simulink model "planLocal_sim"  (R2024a)
settings: Solver=FixedStepDiscrete  StartTime=0.0  StopTime=30  RelTol=1e-3
InitFcn:
  | localPlanSetup
undefined symbols (not defined in the file): n, refPath, tuneableTEBParamsCpp, worldGridLoc, worldMat, worldRes
libraries: roshelperlib x2, simulink x1
settings Model: Creator=cstabile  LastModifiedBy=cstabile
settings SFSimCC: SimTargetLang=C++

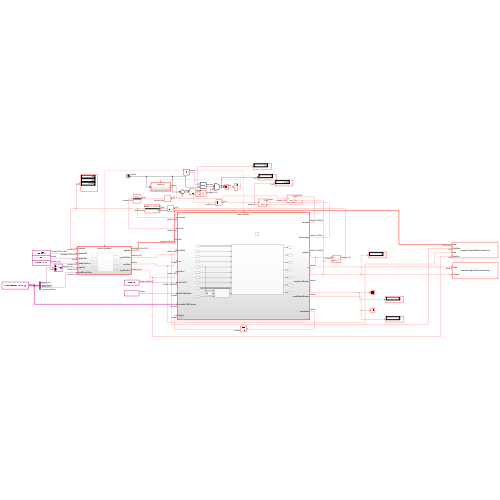
[thumbnail: Simulink's stored preview of the top-level diagram]
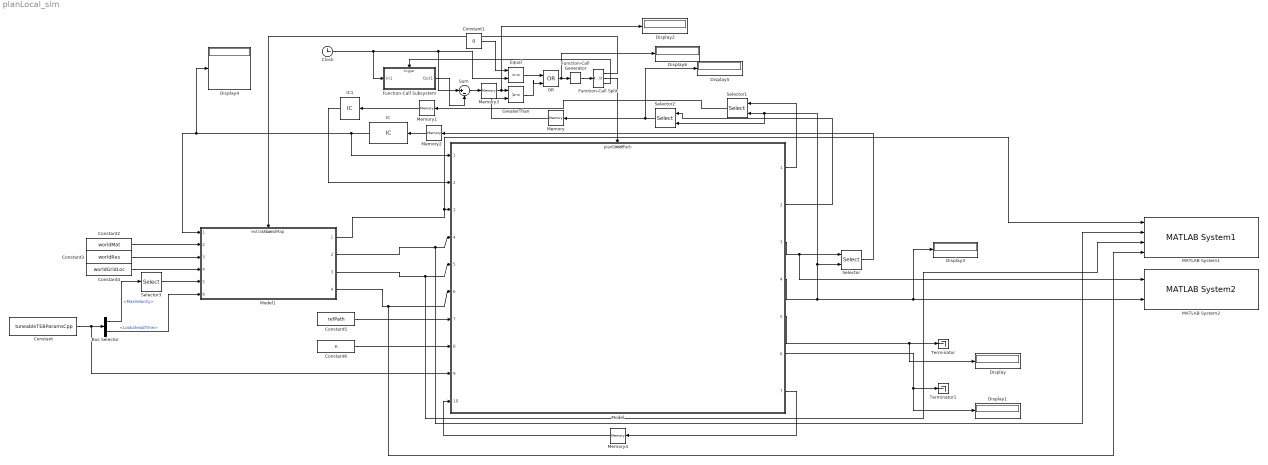
== system planLocal_sim ==
  Bus Selector : BusSelector  OutputSignals=MaxVelocity,LookaheadTime
  Clock : Clock
  Constant : Constant  Value=tuneableTEBParamsCpp  OutDataTypeStr=Bus: teb_bus
  Constant1 : Constant  Value=0
  Constant2 : Constant  Value=worldMat  VectorParams1D=off
  Constant3 : Constant  Value=worldRes
  Constant4 : Constant  Value=worldGridLoc  VectorParams1D=off
  Constant5 : Constant  Value=refPath  VectorParams1D=off
  Constant6 : Constant  Value=n
  Display{,1..6} (7 alike) : Display
  Equal : RelationalOperator  Operator===  OutDataTypeStr=boolean  RndMeth=Simplest  InputSameDT=off
  Function-Call Generator : simulink/Ports & Subsystems/Function-Call Generator  sample_time=1  numberOfIterations=1  DisallowWideOutput=off  ShowEnablePort=on
  Function-Call Split : FunctionCallSplit  IconShape=distinctive  NumOutputPorts=3  OutputPortLayout=default
  Function-Call Subsystem : Subsystem  TreatAsAtomicUnit=on
  GreaterThan : RelationalOperator  OutDataTypeStr=boolean  RndMeth=Simplest  InputSameDT=off
  IC : InitialCondition  Value=refPath(1,:) + [10 10 0]
  IC1 : InitialCondition  Value=[0 0]
  MATLAB System1 : roshelperlib/MATLAB System1  MapType=SDF  IsEgo=on  DisplayVisual=on  SimulateUsing=Interpreted execution
  MATLAB System2 : roshelperlib/MATLAB System2  VisualizationParameters={'k-'}  PlotType=Line  DisplayVisual=on  SimulateUsing=Interpreted execution
  Memory{,1..4} (5 alike) : Memory
  Model : ModelReference  ModelNameDialog=planLocalPath.slx  SimulationMode=Normal  ModelReferenceVersion=1.7  TriggerPortName=function  TriggerPortTriggerType=function-call  TriggerPortStatesWhenEnabling=held
  Model1 : ModelReference  ModelNameDialog=extractLocalMap.slx  SimulationMode=Normal  ModelReferenceVersion=1.0  TriggerPortName=function  TriggerPortTriggerType=function-call  TriggerPortStatesWhenEnabling=held
  OR : Logic  Operator=OR  IconShape=distinctive  AllPortsSameDT=off  OutDataTypeStr=boolean
  Selector : Selector  NumberOfDimensions=2  InputPortWidth=3  IndexOptions=Starting index (port),Select all  Indices=[1 3],1  OutputSizes=1,1
  Selector1 : Selector  NumberOfDimensions=2  InputPortWidth=3  IndexOptions=Starting index (port),Select all  Indices=[1 3],1  OutputSizes=1,1
  Selector2 : Selector  NumberOfDimensions=2  InputPortWidth=3  IndexOptions=Starting index (port),Select all  Indices=[1 3],1  OutputSizes=1,1
  Selector3 : Selector  InputPortWidth=2  IndexOptions=Index vector (dialog)  Indices=1  OutputSizes=1
  Sum : Sum  Inputs=|+-
  Terminator : Terminator
  Terminator1 : Terminator
  wires:
  Clock/1 -> Function-Call Subsystem/1(In1), Sum/1, Equal/2
  Model/2 -> Selector2/1
  GreaterThan/1 -> OR/2
  Equal/1 -> OR/1
  Constant1/1 -> Equal/1
  OR/1 -> Display6/1, Function-Call Generator/1
  Model/3 -> MATLAB System2/1, Selector/1
  Model/4 -> Selector2/2, Selector1/2, Selector/2, MATLAB System2/2, Display3/1
  Selector/1 -> Memory2/1
  Model/1 -> Selector1/1
  Constant2/1 -> Model1/2
  Constant3/1 -> Model1/3
  Constant4/1 -> Model1/4
  Model/5 -> Display/1, Terminator/1
  Model/6 -> Display1/1, Terminator1/1
  Bus Selector/2 -> Model1/6  "<LookaheadTime>"
  Bus Selector/1 -> Selector3/1  "<MaxVelocity>"
  Constant6/1 -> Model/8
  Constant5/1 -> Model/7
  Model1/4 -> MATLAB System1/4, Model/6
  Constant/1 -> Model/9, Bus Selector/1
  Model1/3 -> MATLAB System1/3, Model/5
  Model1/2 -> MATLAB System1/2, Model/4
  Model1/1 -> MATLAB System1/1, Model/3
  Function-Call Split/2 -> Model/Trigger
  IC1/1 -> Model/2
  IC/1 -> Display4/1, Model1/1, Model/1
  Selector1/1 -> Memory1/1
  Selector3/1 -> Model1/5
  Function-Call Generator/1 -> Function-Call Split/1
  Selector2/1 -> Display5/1, Memory/1
  Function-Call Split/1 -> Model1/Trigger
  Memory/1 -> GreaterThan/2
  Memory1/1 -> IC1/1
  Memory2/1 -> IC/1
  Function-Call Split/3 -> Function-Call Subsystem/Trigger
  Function-Call Subsystem/1(Out1) -> Sum/2
  Sum/1 -> Memory3/1
  Memory3/1 -> Display2/1, GreaterThan/1
  Model/7 -> Memory4/1
  Memory4/1 -> Model/10

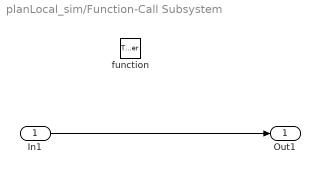
== system planLocal_sim/Function-Call Subsystem ==
  In1 : Inport
  function : TriggerPort  TriggerType=function-call  VariantControl=(inherit)
  Out1 : Outport
  wires:
  In1/1 -> Out1/1
